simulink model "TestforElasticCtrl"  (R2019b)
settings: Solver=VariableStepAuto  StartTime=0.0  StopTime=10.0  RelTol=1e-6  AbsTol=1e-6
undefined symbols (not defined in the file or in its folder): Continuous, Time
libraries: dsparch4 x3, ctrlSharedLib x1
settings Model: Creator=19398  LastModifiedBy=19398

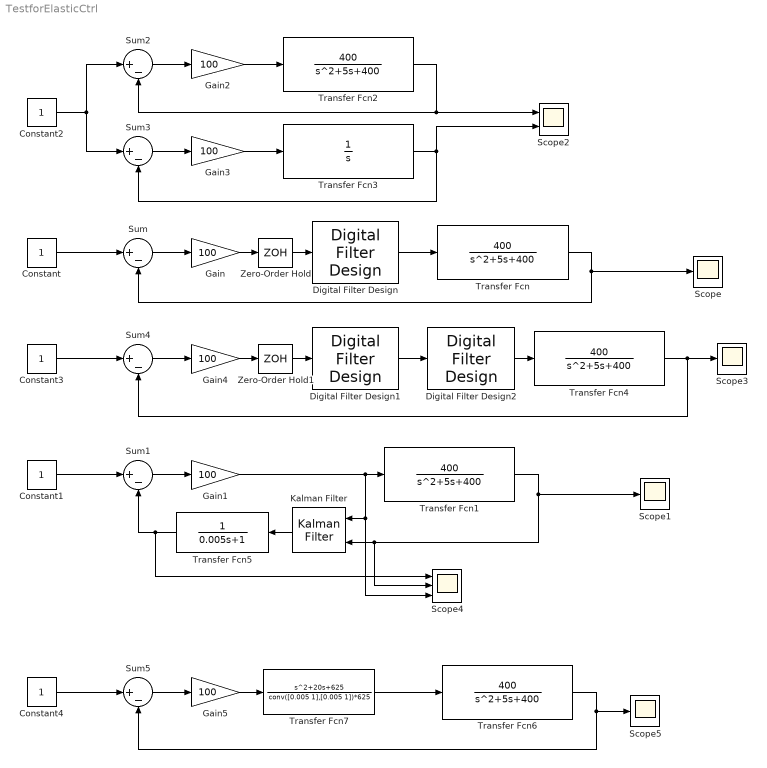
== system TestforElasticCtrl ==
  Constant{,1..4} (5 alike) : Constant
  Digital Filter Design : dsparch4/Digital Filter Design  mwdsp_browser_bugfix_var=off
  Digital Filter Design1 : dsparch4/Digital Filter Design  mwdsp_browser_bugfix_var=off
  Digital Filter Design2 : dsparch4/Digital Filter Design  mwdsp_browser_bugfix_var=off
  Gain{,1..5} (6 alike) : Gain  Gain=100
  Kalman Filter : ctrlSharedLib/Kalman Filter  TimeDomain=Continuous-Time  UseCurrentEstimator=on  ModelSource=Individual A, B, C, D matrices  ModelSourceVariable=ss(0.95,1,1,0,1)  A=0  B=1  C=1  D=0  NumberOfStates=1  NumberOfInputs=1  NumberOfOutputs=1  InitialEstimateSource=Dialog  X0=0  P0=10  UseK=off  UseGH=off  NumberOfProcessNoiseInputs=1  G=1  TimeInvariantG=on  H=0  TimeInvariantH=on  Q=0.5  TimeInvariantQ=on  R=1  TimeInvariantR=on  N=0  TimeInvariantN=on  AddInputPort=on  AddEnablePort=off  OutputEstimatedY=off  OutputP=off  Ts=-1
      settings: SourceProductBaseCode=CT
  Scope{,1,3,5} (4 alike) : Scope
  Scope2 : Scope  NumInputPorts=2
  Scope4 : Scope  NumInputPorts=3
  Sum{,1..5} (6 alike) : Sum  Inputs=|+-
  Transfer Fcn{,1..2,4,6} (5 alike) : TransferFcn  Numerator=[400]  Denominator=[1 5 400]
  Transfer Fcn3 : TransferFcn  Denominator=[1 0]
  Transfer Fcn5 : TransferFcn  Denominator=[0.005 1]
  Transfer Fcn7 : TransferFcn  Numerator=[1 20 625]  Denominator=conv([0.005 1],[0.005 1])*625
  Zero-Order Hold : ZeroOrderHold  SampleTime=0.002
  Zero-Order Hold1 : ZeroOrderHold  SampleTime=0.005
  wires:
  Constant/1 -> Sum/1
  Sum/1 -> Gain/1
  Gain/1 -> Zero-Order Hold/1
  Transfer Fcn/1 -> Scope/1, Sum/2
  Digital Filter Design/1 -> Transfer Fcn/1
  Zero-Order Hold/1 -> Digital Filter Design/1
  Sum1/1 -> Gain1/1
  Gain1/1 -> Scope4/3, Kalman Filter/1, Transfer Fcn1/1
  Constant1/1 -> Sum1/1
  Transfer Fcn1/1 -> Scope1/1, Scope4/2, Kalman Filter/2
  Sum2/1 -> Gain2/1
  Gain2/1 -> Transfer Fcn2/1
  Constant2/1 -> Sum2/1, Sum3/1
  Transfer Fcn2/1 -> Sum2/2, Scope2/1
  Kalman Filter/1 -> Transfer Fcn5/1
  Transfer Fcn5/1 -> Sum1/2, Scope4/1
  Gain3/1 -> Transfer Fcn3/1
  Transfer Fcn3/1 -> Sum3/2, Scope2/2
  Sum3/1 -> Gain3/1
  Constant3/1 -> Sum4/1
  Gain4/1 -> Zero-Order Hold1/1
  Sum4/1 -> Gain4/1
  Transfer Fcn4/1 -> Sum4/2, Scope3/1
  Digital Filter Design2/1 -> Transfer Fcn4/1
  Zero-Order Hold1/1 -> Digital Filter Design1/1
  Digital Filter Design1/1 -> Digital Filter Design2/1
  Transfer Fcn6/1 -> Sum5/2, Scope5/1
  Constant4/1 -> Sum5/1
  Gain5/1 -> Transfer Fcn7/1
  Sum5/1 -> Gain5/1
  Transfer Fcn7/1 -> Transfer Fcn6/1
